simulink model "Helicopter_comparison"  (R2018a)
settings: Solver=VariableStepAuto  StartTime=0.0  StopTime=inf  RelTol=1e-3
values from neighbouring files (symbols this model uses):
  Bp = 0.01    [Helicopter_Values.m]
  By = 0.08    [Helicopter_Values.m]
  g = 9.81    [Helicopter_Values.m]
  jeqp = 0.0172    [Helicopter_Values.m]
  jeqy = 0.021    [Helicopter_Values.m]
  kpp = 0.0556    [Helicopter_Values.m]
  kpy = 0.005    [Helicopter_Values.m]
  kyp = 0.15    [Helicopter_Values.m]
  kyy = 0.21084    [Helicopter_Values.m]
  lcm = 0.015    [Helicopter_Values.m]
  mheli = 0.479    [Helicopter_Values.m]
  Vmp_op = (kyy*mheli*g*cos(p_r_op)*lcm)/(kyy*kpp -kyp*kpy)    [Helicopter_Values.m]
  Vmy_op = kyp*Vmp_op/kyy    [Helicopter_Values.m]
libraries: realtime_pacer_lib x1
settings Model: Creator=pacoa  LastModifiedBy=pacoa

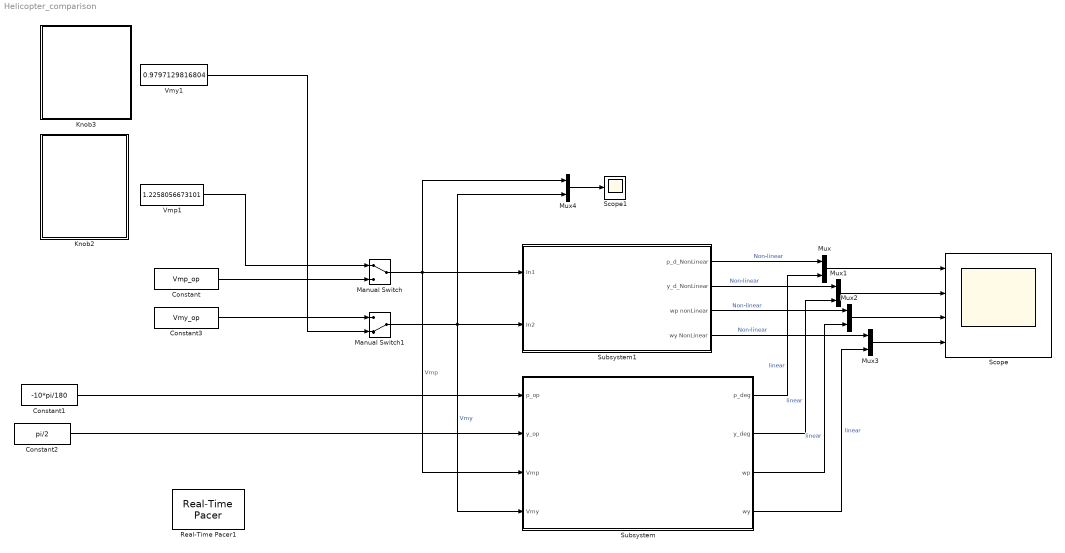
== system Helicopter_comparison ==
  Constant : Constant  Value=Vmp_op
  Constant1 : Constant  Value=-10*pi/180
  Constant2 : Constant  Value=pi/2
  Constant3 : Constant  Value=Vmy_op
  Knob2 : Subsystem  DialogController=hmiCreateDDGDialog  IsWebBlock=on  mask(MWDashboardBlock){webBlockId=2947dbe9-c983-48e5-a0e7-08dc830ec4db, webBlockType=continuousknob, ShowInLibBrowser=on, ShowInitialText=on, HMISrcModelName=Helicopter_comparison}
      mask prompts: webBlockId "WebBlock Id"; webBlockType "WebBlock Type"; HMISrcModelName "Source Model"
      mask help: SimulinkHMI:dialogs:ContinuousKnobDialogDesc
      mask Help: helpview([docroot '/mapfiles/simulink.map'], 'hmi_knob')
      mask Display:
      | if strcmp(get_param(bdroot(gcb),'BlockDiagramType'), 'library')
      |     image([(matlabroot) '/toolbox/simulink/hmi/icons/ContinuousKnob.png']);
      | end
  Knob3 : Subsystem  DialogController=hmiCreateDDGDialog  IsWebBlock=on  mask(MWDashboardBlock){webBlockId=c647893d-3700-434c-8494-02a4b62e6e85, webBlockType=continuousknob, ShowInLibBrowser=on, ShowInitialText=on, HMISrcModelName=Helicopter_comparison}
      mask prompts: webBlockId "WebBlock Id"; webBlockType "WebBlock Type"; HMISrcModelName "Source Model"
      mask help: SimulinkHMI:dialogs:ContinuousKnobDialogDesc
      mask Help: helpview([docroot '/mapfiles/simulink.map'], 'hmi_knob')
      mask Display:
      | if strcmp(get_param(bdroot(gcb),'BlockDiagramType'), 'library')
      |     image([(matlabroot) '/toolbox/simulink/hmi/icons/ContinuousKnob.png']);
      | end
  Manual Switch : ManualSwitch
  Manual Switch1 : ManualSwitch  CurrentSetting=0
  Mux{,1..4} (5 alike) : Mux  Inputs=2
  Real-Time Pacer1 : realtime_pacer_lib/Real-Time Pacer  simTimePerRealTime=10
  Scope : Scope  NumInputPorts=4
  Scope1 : Scope
  Subsystem : Subsystem
  Subsystem1 : Subsystem
  Vmp1 : Constant  Value=1.2258056673101
  Vmy1 : Constant  Value=0.9797129816804
  wires:
  Constant3/1 -> Manual Switch1/1
  Constant2/1 -> Subsystem/2(y_op)
  Constant1/1 -> Subsystem/1(p_op)
  Constant/1 -> Manual Switch/2
  Manual Switch/1 -> Mux4/1, Subsystem1/1(In1), Subsystem/3(Vmp)  "Vmp"
  Manual Switch1/1 -> Mux4/2, Subsystem1/2(In2), Subsystem/4(Vmy)  "Vmy"
  Vmp1/1 -> Manual Switch/1
  Vmy1/1 -> Manual Switch1/2
  Subsystem/1(p_deg) -> Mux/2  "linear"
  Subsystem1/1(p_d_NonLinear) -> Mux/1  "Non-linear"
  Subsystem/2(y_deg) -> Mux1/2  "linear"
  Subsystem/3(wp) -> Mux2/2  "linear"
  Subsystem1/4(wy NonLinear) -> Mux3/1  "Non-linear"
  Subsystem/4(wy) -> Mux3/2  "linear"
  Mux1/1 -> Scope/2
  Mux/1 -> Scope/1
  Mux2/1 -> Scope/3
  Mux3/1 -> Scope/4
  Subsystem1/3(wp nonLinear) -> Mux2/1  "Non-linear"
  Subsystem1/2(y_d_NonLinear) -> Mux1/1  "Non-linear"
  Mux4/1 -> Scope1/1

== system Helicopter_comparison/Knob2 ==

== system Helicopter_comparison/Knob3 ==

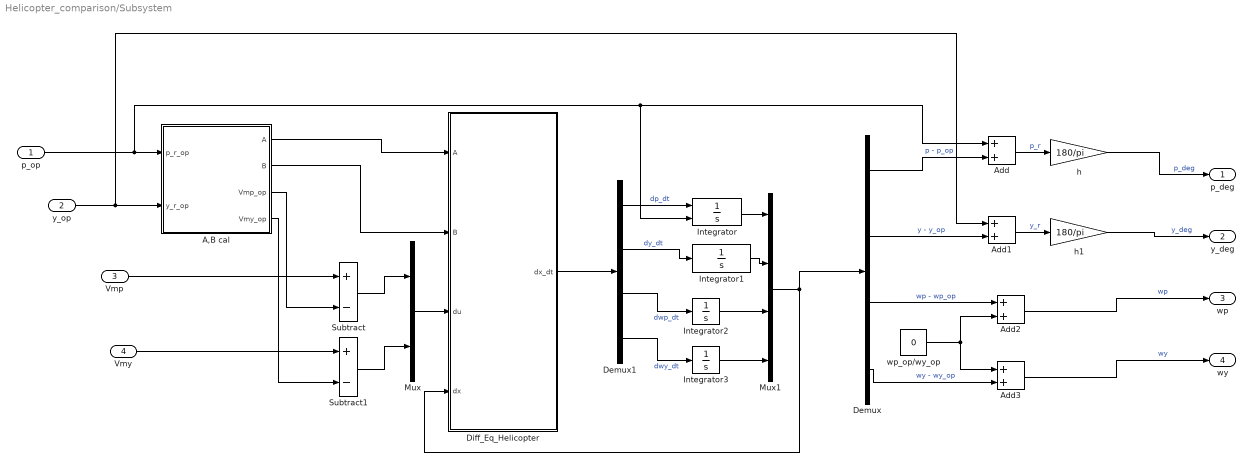
== system Helicopter_comparison/Subsystem ==
  p_op : Inport
  y_op : Inport  Port=2
  Vmp : Inport  Port=3
  Vmy : Inport  Port=4
  A,B cal : MATLAB Function  TreatAsAtomicUnit=on
  Add{,1..3} (4 alike) : Sum
  Demux : Demux
  Demux1 : Demux
  Diff_Eq_Helicopter : MATLAB Function  TreatAsAtomicUnit=on
  Integrator : Integrator  InitialConditionSource=external  InitialCondition=-10*pi/180  LimitOutput=on  UpperSaturationLimit=pi/4 - (-10*pi/180)  LowerSaturationLimit=-pi/4 - (-10*pi/180)
  Integrator1 : Integrator  LimitOutput=on  UpperSaturationLimit=pi - (pi/2)  LowerSaturationLimit=0 - (pi/2)
  Integrator2 : Integrator  UpperSaturationLimit=pi
  Integrator3 : Integrator
  Mux : Mux  Inputs=2
  Mux1 : Mux
  Subtract : Sum  Inputs=+-
  Subtract1 : Sum  Inputs=+-
  h : Gain  Gain=180/pi
  h1 : Gain  Gain=180/pi
  wp_op/wy_op : Constant  Value=0
  p_deg : Outport
  y_deg : Outport  Port=2
  wp : Outport  Port=3
  wy : Outport  Port=4
  wires:
  Vmy/1 -> Subtract1/1
  Integrator/1 -> Mux1/1
  A,B cal/4(Vmy_op) -> Subtract1/2
  A,B cal/2(B) -> Diff_Eq_Helicopter/2(B)
  Add3/1 -> wy/1  "wy"
  Demux1/1 -> Integrator/1  "dp_dt"
  p_op/1 -> A,B cal/1(p_r_op), Integrator/2, Add/1
  Demux1/2 -> Integrator1/1  "dy_dt"
  Integrator3/1 -> Mux1/4
  Demux/3 -> Add2/1  "wp - wp_op"
  A,B cal/1(A) -> Diff_Eq_Helicopter/1(A)
  Mux/1 -> Diff_Eq_Helicopter/3(du)
  Add1/1 -> h1/1  "y_r"
  Add/1 -> h/1  "p_r"
  y_op/1 -> Add1/1, A,B cal/2(y_r_op)
  Subtract/1 -> Mux/1
  Diff_Eq_Helicopter/1(dx_dt) -> Demux1/1
  Mux1/1 -> Demux/1, Diff_Eq_Helicopter/4(dx)
  Demux/4 -> Add3/2  "wy - wy_op"
  Demux1/4 -> Integrator3/1  "dwy_dt"
  Vmp/1 -> Subtract/1
  Subtract1/1 -> Mux/2
  h/1 -> p_deg/1  "p_deg"
  Integrator2/1 -> Mux1/3
  A,B cal/3(Vmp_op) -> Subtract/2
  wp_op/wy_op/1 -> Add2/2, Add3/1
  Demux1/3 -> Integrator2/1  "dwp_dt"
  Demux/1 -> Add/2  "p - p_op"
  Integrator1/1 -> Mux1/2
  Demux/2 -> Add1/2  "y - y_op"
  Add2/1 -> wp/1  "wp"
  h1/1 -> y_deg/1  "y_deg"

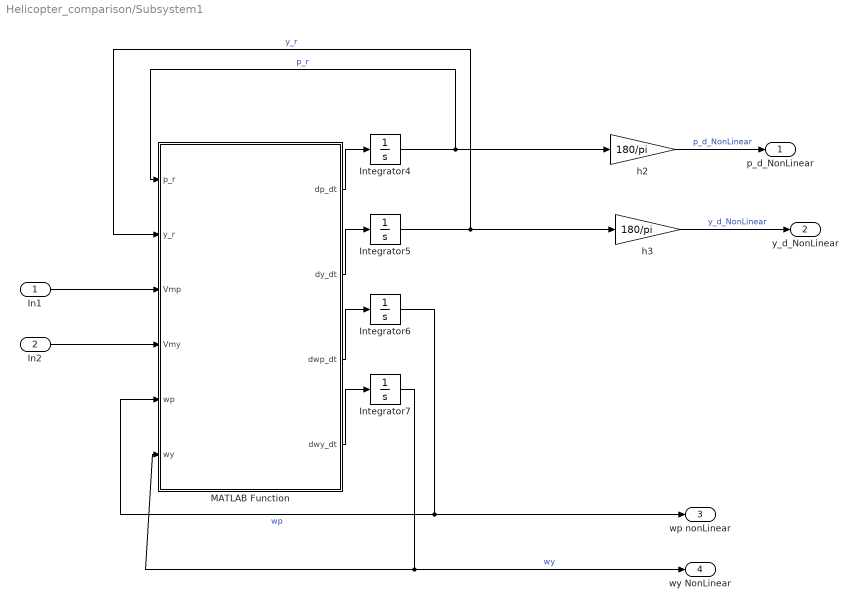
== system Helicopter_comparison/Subsystem1 ==
  In1 : Inport
  In2 : Inport  Port=2
  Integrator4 : Integrator  InitialCondition=-10*pi/180  LimitOutput=on  UpperSaturationLimit=pi/4  LowerSaturationLimit=-pi/4
  Integrator5 : Integrator  InitialCondition=pi/2  LimitOutput=on  UpperSaturationLimit=pi  LowerSaturationLimit=0
  Integrator6 : Integrator
  Integrator7 : Integrator
  MATLAB Function : MATLAB Function  TreatAsAtomicUnit=on
  h2 : Gain  Gain=180/pi
  h3 : Gain  Gain=180/pi
  p_d_NonLinear : Outport
  y_d_NonLinear : Outport  Port=2
  wp nonLinear : Outport  Port=3
  wy NonLinear : Outport  Port=4
  wires:
  In1/1 -> MATLAB Function/3(Vmp)
  Integrator5/1 -> h3/1, MATLAB Function/2(y_r)  "y_r"
  MATLAB Function/3(dwp_dt) -> Integrator6/1
  Integrator7/1 -> wy NonLinear/1, MATLAB Function/6(wy)  "wy"
  MATLAB Function/2(dy_dt) -> Integrator5/1
  MATLAB Function/4(dwy_dt) -> Integrator7/1
  h2/1 -> p_d_NonLinear/1  "p_d_NonLinear"
  MATLAB Function/1(dp_dt) -> Integrator4/1
  Integrator6/1 -> MATLAB Function/5(wp), wp nonLinear/1  "wp"
  Integrator4/1 -> h2/1, MATLAB Function/1(p_r)  "p_r"
  In2/1 -> MATLAB Function/4(Vmy)
  h3/1 -> y_d_NonLinear/1  "y_d_NonLinear"

== matlab function Helicopter_comparison/Subsystem/Diff_Eq_Helicopter ==
  data: A input; B input; du input size=[2 1]; dx_dt output; dx input size=[4 1]
function dx_dt = fcn(A,B,du,dx)

dx_dt =A*dx + B*(du);

== matlab function Helicopter_comparison/Subsystem/A,B cal ==
  data: p_r_op input; A output; B output; y_r_op input; lcm parameter; mheli parameter; jeqp parameter; jeqy parameter; g parameter; kpp parameter; kyy parameter; kyp parameter; Bp parameter; By parameter; kpy parameter; Vmp_op output; Vmy_op output
function [A,B,Vmp_op,Vmy_op] = fcn(p_r_op,y_r_op, lcm, mheli, jeqp, jeqy, g, kpp, kyy, kyp, Bp, By, kpy)



Vmp_op = (kyy*mheli*g*cos(p_r_op)*lcm)/(kyy*kpp -kyp*kpy);
Vmy_op = kyp*Vmp_op/kyy;
%% A and B
%A
A1_3 = 1;

A2_4 = 1;

A3_1 = mheli*g*lcm*sin(p_r_op)/(jeqp +mheli*lcm*lcm);
A3_3 = -Bp/(jeqp +mheli*lcm*lcm);

A4_1_n = (kyp*Vmp_op -kyy*Vmy_op)*2*mheli*lcm*lcm*sin(p_r_op)*cos(p_r_op);
A4_1_d = (jeqy +mheli*cos(p_r_op)*cos(p_r_op)*lcm*lcm)^2;
A4_1 = A4_1_n/A4_1_d;

A4_4_d = (jeqy +mheli*cos(p_r_op)*cos(p_r_op)*lcm*lcm);
A4_4 = -By/A4_4_d;

A1 = [0, 0, A1_3, 0];
A2 = [0, 0, 0, A2_4];
A3 = [A3_1, 0, A3_3, 0];
A4 = [A4_1, 0, 0, A4_4];

A =[A1;A2;A3;A4];

%B
B3_d = (jeqp +mheli*lcm*lcm);
B3_1 = kpp/(B3_d);
B3_2 = -kpy/(B3_d);
B4_d = jeqy +mheli*cos(p_r_op)*cos(p_r_op)*lcm*lcm;
B4_1 = kyp/B4_d;
B4_2 = -kyy/B4_d;

B1 = [0,0];
B2 = [0,0];
B3 = [B3_1,B3_2];
B4 = [B4_1,B4_2];

B = [B1;B2;B3;B4];

== matlab function Helicopter_comparison/Subsystem1/MATLAB Function ==
  data: p_r input; y_r input; Vmp input; Vmy input; wp input; dp_dt output size=[1 1]; wy input; dy_dt output size=[1 1]; dwp_dt output size=[1 1]; dwy_dt output size=[1 1]; lcm parameter; mheli parameter; jeqp parameter; jeqy parameter; g parameter; kpp parameter; kyy parameter; kyp parameter; Bp parameter; By parameter; kpy parameter
function [dp_dt, dy_dt, dwp_dt, dwy_dt]= fcn(p_r,y_r,Vmp, Vmy,wp,wy, lcm, mheli, jeqp, jeqy, g, kpp, kyy,kyp, Bp, By, kpy)
  %%Parameters
%   
%   Bp,
%   By,
%   g,
%   kpp,
%   kyp,
%   kyy,
%   kpy,
%   mheli,
%   lcm,
%   jeqp,
%   jeqy,
  

%%
   dp_dt = wp;
   dy_dt = wy;
   
   %%
   dwp_dt_n1 = (kpp*Vmp);
   dwp_dt_n2 = (kpy*Vmy);
   dwp_dt_n3 = (Bp*wp+ (mheli*(wy.^2)*sin(p_r)*(lcm^2)*cos(p_r) + (mheli*g*cos(p_r)*lcm)));
   
   dwp_dt_d = (jeqp + mheli*(lcm^2));
   
   dwp_dt = (dwp_dt_n1 -dwp_dt_n2 - dwp_dt_n3)/(dwp_dt_d);
   
   %%
   dwy_dt_n1 = kyp*Vmp;
   dwy_dt_n2 = kyy*Vmy;
   dwy_dt_n3 = 2*mheli*(wy)*sin(p_r)*(lcm^2)*cos(p_r)*wp;
   dwy_dt_n4 = By*wy;
   
   dwy_dt_d = jeqy + mheli*((cos(p_r))^2)*(lcm^2);
   
   dwy_dt = (dwy_dt_n1 - dwy_dt_n2 + dwy_dt_n3 -dwy_dt_n4)/(dwy_dt_d);
